simulink model "dataFiltering"  (Simulink 8.0)
settings: Solver=ode3  StartTime=0.0  StopTime=Td  FixedStep=Ts  RelTol=1e-3
undefined symbols (not defined in the file or in its folder): filtOrder, Ts
libraries: dsparch4 x1
settings Model: Creator=esobha  LastModifiedBy=esobha
settings DataIOCC: SignalLoggingSaveFormat=ModelDataLogs
settings DebuggingCC: FcnCallInpInsideContextMsg=UseLocalSettings
settings GRTTargetCC: CombineOutputUpdateFcns=off  GRTInterface=on

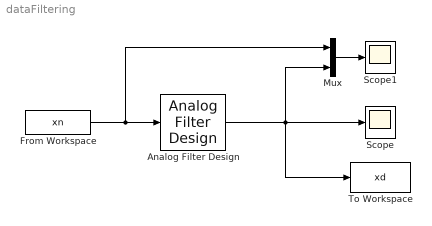
== system dataFiltering ==
  Analog Filter Design : dsparch4/Analog Filter Design  method=Butterworth  filttype=Lowpass  N=filtOrder  Wlo=filtBW  Whi=80  Rp=2  Rs=60
  From Workspace : FromWorkspace  VariableName=xn  SampleTime=Ts
  Mux : Mux  Inputs=2
  Scope : Scope
  Scope1 : Scope
  To Workspace : ToWorkspace  VariableName=xd  SampleTime=Ts
  wires:
  From Workspace/1 -> Analog Filter Design/1, Mux/1
  Analog Filter Design/1 -> Scope/1, Mux/2, To Workspace/1
  Mux/1 -> Scope1/1
